simulink model "ReferenceGenerator"  (R2018a)
settings: Solver=VariableStepAuto  StartTime=0.0  StopTime=10.0  RelTol=1e-3
PreLoadFcn:
  | modelDir = fileparts(get_param(bdroot, 'FileName'));
  | addpath(fullfile(modelDir,'../Parameters'));
  | addpath(fullfile(modelDir,'subsystems'));
  | 
  | Parameters_General
  | Parameters_Simulation
  | Parameters_Controllers
InitFcn:
  | Parameters_General
  | Parameters_Simulation
  | Parameters_Controllers
undefined symbols (not defined in the file or in its folder): chirp_amplitude_deg, f_sine, omega_b_ref, q_ref, rate_chirp, ReferenceMode, roll_sine_amplitude_deg, Ts
libraries: simulink x1
settings Model: Creator=Thomas  LastModifiedBy=Thomas

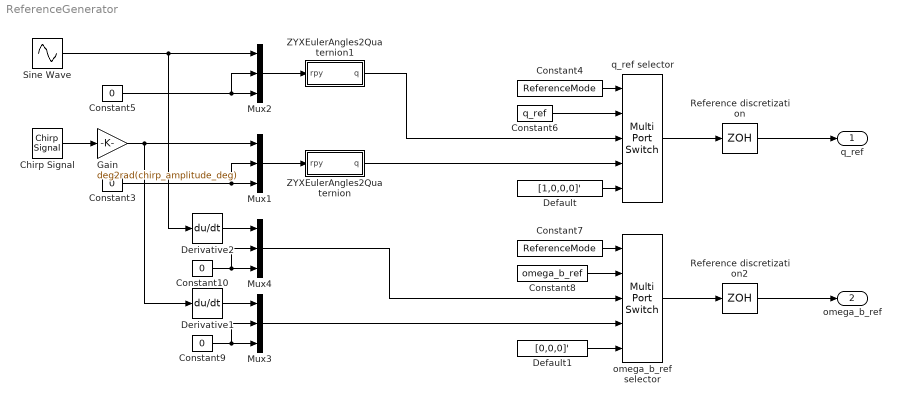
== system ReferenceGenerator ==
  Chirp Signal : simulink/Sources/Chirp Signal  f1=f0_chirp  T=100  f2=100*rate_chirp
  Constant{3,5,9..10} (4 alike) : Constant  Value=0
  Constant4 : Constant  Value=ReferenceMode
  Constant6 : Constant  Value=q_ref
  Constant7 : Constant  Value=ReferenceMode
  Constant8 : Constant  Value=omega_b_ref
  Default : Constant  Value=[1,0,0,0]'
  Default1 : Constant  Value=[0,0,0]'
  Derivative1 : Derivative
  Derivative2 : Derivative
  Gain : Gain  Gain=deg2rad(chirp_amplitude_deg)
  Mux{1..4} (4 alike) : Mux  Inputs=3
  Reference discretization : ZeroOrderHold  SampleTime=Ts
  Reference discretization2 : ZeroOrderHold  SampleTime=Ts
  Sine Wave : Sin  Amplitude=deg2rad(roll_sine_amplitude_deg)  Frequency=2*pi*f_sine  SampleTime=0
  ZYXEulerAngles2Quaternion : MATLAB Function  TreatAsAtomicUnit=on
  ZYXEulerAngles2Quaternion1 : MATLAB Function  TreatAsAtomicUnit=on
  omega_b_ref selector : MultiPortSwitch  DataPortOrder=Zero-based contiguous  DataPortForDefault=Additional data port  zeroidx=on
  q_ref selector : MultiPortSwitch  DataPortOrder=Zero-based contiguous  DataPortForDefault=Additional data port  zeroidx=on
  q_ref : Outport
  omega_b_ref : Outport  Port=2
  wires:
  Constant4/1 -> q_ref selector/1
  Constant5/1 -> Mux2/2, Mux2/3
  Constant6/1 -> q_ref selector/2
  Constant8/1 -> omega_b_ref selector/2
  Constant7/1 -> omega_b_ref selector/1
  Gain/1 -> Derivative1/1, Mux1/1
  Mux1/1 -> ZYXEulerAngles2Quaternion/1(rpy)
  Mux2/1 -> ZYXEulerAngles2Quaternion1/1(rpy)
  ZYXEulerAngles2Quaternion1/1(q) -> q_ref selector/3
  Mux4/1 -> omega_b_ref selector/3
  ZYXEulerAngles2Quaternion/1(q) -> q_ref selector/4
  Chirp Signal/1 -> Gain/1
  Constant10/1 -> Mux4/2, Mux4/3
  omega_b_ref selector/1 -> Reference discretization2/1
  Mux3/1 -> omega_b_ref selector/4
  Default/1 -> q_ref selector/5
  Sine Wave/1 -> Derivative2/1, Mux2/1
  Constant3/1 -> Mux1/2, Mux1/3
  Derivative2/1 -> Mux4/1
  Derivative1/1 -> Mux3/1
  Constant9/1 -> Mux3/2, Mux3/3
  q_ref selector/1 -> Reference discretization/1
  Default1/1 -> omega_b_ref selector/5
  Reference discretization/1 -> q_ref/1
  Reference discretization2/1 -> omega_b_ref/1

== matlab function ReferenceGenerator/ZYXEulerAngles2Quaternion ==
  data: rpy input size=3; q output size=4
function q = ZYXEulerAngles2Quaternion(rpy)
    q = ZYXEulerAngles2Quaternion(rpy);
end

== matlab function ReferenceGenerator/ZYXEulerAngles2Quaternion1 ==
  data: rpy input size=3; q output size=4
function q = ZYXEulerAngles2Quaternion(rpy)
    q = ZYXEulerAngles2Quaternion(rpy);
end
